simulink model "Train5"  (R2020b)
settings: Solver=VariableStepAuto  StartTime=0.0  StopTime=10.0  RelTol=1e-3
model workspace (MAT data in the model file):
  c = 8
  k = 0.1
undefined symbols (not defined in the file): M_1, M_2, M_3, M_4, M_5, X0_2, X0_3, X0_4, X0_5
settings Model: OrderedModelArguments=off  Creator=zhenya  LastModifiedBy=zhenya

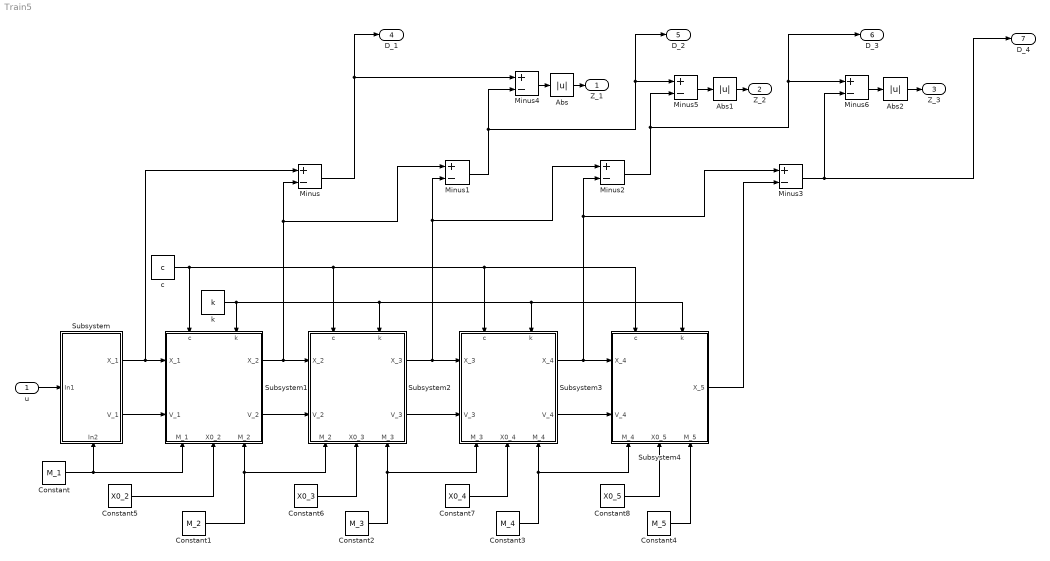
== system Train5 ==
  u : Inport
  Abs : Abs
  Abs1 : Abs
  Abs2 : Abs
  Constant : Constant  Value=M_1
  Constant1 : Constant  Value=M_2
  Constant2 : Constant  Value=M_3
  Constant3 : Constant  Value=M_4
  Constant4 : Constant  Value=M_5
  Constant5 : Constant  Value=X0_2
  Constant6 : Constant  Value=X0_3
  Constant7 : Constant  Value=X0_4
  Constant8 : Constant  Value=X0_5
  Minus{,1..6} (7 alike) : Sum  Inputs=+-
  Subsystem : Subsystem
      settings: PortSchema="{\"entries\":[{\"content\":{\"sides\":[{\"content\":{\"connectorIds\":[\"In1\"]},\"type\":\"ConnectorPlacement.EquallySpacedRectSide\",\"uuid\":\"34ca8425-fccb-4da0-be07-954015c86f74\"},{\"content\":{\"connectorIds\":[\"Out1\",\"Out2\"],\"side\":\"RIGHT\"},\"type\":\"ConnectorPlacement.EquallySpacedRectSide\",\"uuid\":\"a4a70c44-d99b-4f2f-bcd7-1dd85156dc1f\"},{\"content\":{\"connectorIds\":[],\"side\":\"TOP\"},\"type\":\"ConnectorPlacement.EquallySpacedRectSide\",\"uuid\":\"14968497-3b66-4f95-885e-db1a1d92cb6f\"},{\"content\":{\"connectorIds\":[\"In2\"],\"side\":\"BOTTOM\"},\"type\":\"ConnectorPlacement.EquallySpacedRectSide\",\"uuid\":\"7000d41a-f478-4b38-bf4d-e27f7f915c37\"},{\"content\":{\"connectorIds\":[],\"side\":\"HIDDEN\"},\"type\":\"ConnectorPlacement.EquallySpacedRectSide\",\"uuid\":\"79f1d2cd-3fc8-42f6-ae8b-07eaf6f97827\"}]},\"type\":\"ConnectorPlacement.EquallySpacedConnector\",\"uuid\":\"0ff0aa4c-6fa5-4dba-bb7c-396d165f33e0\"}],\"packageUris\":[\"http://schema.mathworks.com/mf0/Connector/R2020b\"],\"version\":\"1.0\"}"
  Subsystem1 : Subsystem
      settings: PortSchema="{\"entries\":[{\"content\":{\"sides\":[{\"content\":{\"connectorIds\":[\"In1\",\"In2\"]},\"type\":\"ConnectorPlacement.EquallySpacedRectSide\",\"uuid\":\"638557b6-12c9-401f-951d-5f98dd7903cc\"},{\"content\":{\"connectorIds\":[\"Out1\",\"Out2\"],\"side\":\"RIGHT\"},\"type\":\"ConnectorPlacement.EquallySpacedRectSide\",\"uuid\":\"d2d0712b-4eed-449a-bee8-cfe81cb0f76e\"},{\"content\":{\"connectorIds\":[\"In3\",\"In4\"],\"side\":\"TOP\"},\"type\":\"ConnectorPlacement.EquallySpacedRectSide\",\"uuid\":\"1558c73d-fb4f-4eb2-a0a5-81154d1cf643\"},{\"content\":{\"connectorIds\":[\"In5\",\"In6\",\"In7\"],\"side\":\"BOTTOM\"},\"type\":\"ConnectorPlacement.EquallySpacedRectSide\",\"uuid\":\"3af12584-476c-4d41-9154-a12458e629fd\"},{\"content\":{\"connectorIds\":[],\"side\":\"HIDDEN\"},\"type\":\"ConnectorPlacement.EquallySpacedRectSide\",\"uuid\":\"cdf596f7-1fd7-4460-9128-df53dc6c9dd6\"}]},\"type\":\"ConnectorPlacement.EquallySpacedConnector\",\"uuid\":\"66e3da69-735a-4605-b465-2e84808dff46\"}],\"packageUris\":[\"http://schema.mathworks.com/mf0/Connector/R2020b\"],\"version\":\"1.0\"}"
  Subsystem2 : Subsystem
      settings: PortSchema="{\"entries\":[{\"content\":{\"sides\":[{\"content\":{\"connectorIds\":[\"In1\",\"In2\"]},\"type\":\"ConnectorPlacement.EquallySpacedRectSide\",\"uuid\":\"638557b6-12c9-401f-951d-5f98dd7903cc\"},{\"content\":{\"connectorIds\":[\"Out1\",\"Out2\"],\"side\":\"RIGHT\"},\"type\":\"ConnectorPlacement.EquallySpacedRectSide\",\"uuid\":\"d2d0712b-4eed-449a-bee8-cfe81cb0f76e\"},{\"content\":{\"connectorIds\":[\"In3\",\"In4\"],\"side\":\"TOP\"},\"type\":\"ConnectorPlacement.EquallySpacedRectSide\",\"uuid\":\"1558c73d-fb4f-4eb2-a0a5-81154d1cf643\"},{\"content\":{\"connectorIds\":[\"In5\",\"In6\",\"In7\"],\"side\":\"BOTTOM\"},\"type\":\"ConnectorPlacement.EquallySpacedRectSide\",\"uuid\":\"3af12584-476c-4d41-9154-a12458e629fd\"},{\"content\":{\"connectorIds\":[],\"side\":\"HIDDEN\"},\"type\":\"ConnectorPlacement.EquallySpacedRectSide\",\"uuid\":\"cdf596f7-1fd7-4460-9128-df53dc6c9dd6\"}]},\"type\":\"ConnectorPlacement.EquallySpacedConnector\",\"uuid\":\"66e3da69-735a-4605-b465-2e84808dff46\"}],\"packageUris\":[\"http://schema.mathworks.com/mf0/Connector/R2020b\"],\"version\":\"1.0\"}"
  Subsystem3 : Subsystem
      settings: PortSchema="{\"entries\":[{\"content\":{\"sides\":[{\"content\":{\"connectorIds\":[\"In1\",\"In2\"]},\"type\":\"ConnectorPlacement.EquallySpacedRectSide\",\"uuid\":\"638557b6-12c9-401f-951d-5f98dd7903cc\"},{\"content\":{\"connectorIds\":[\"Out1\",\"Out2\"],\"side\":\"RIGHT\"},\"type\":\"ConnectorPlacement.EquallySpacedRectSide\",\"uuid\":\"d2d0712b-4eed-449a-bee8-cfe81cb0f76e\"},{\"content\":{\"connectorIds\":[\"In3\",\"In4\"],\"side\":\"TOP\"},\"type\":\"ConnectorPlacement.EquallySpacedRectSide\",\"uuid\":\"1558c73d-fb4f-4eb2-a0a5-81154d1cf643\"},{\"content\":{\"connectorIds\":[\"In5\",\"In6\",\"In7\"],\"side\":\"BOTTOM\"},\"type\":\"ConnectorPlacement.EquallySpacedRectSide\",\"uuid\":\"3af12584-476c-4d41-9154-a12458e629fd\"},{\"content\":{\"connectorIds\":[],\"side\":\"HIDDEN\"},\"type\":\"ConnectorPlacement.EquallySpacedRectSide\",\"uuid\":\"cdf596f7-1fd7-4460-9128-df53dc6c9dd6\"}]},\"type\":\"ConnectorPlacement.EquallySpacedConnector\",\"uuid\":\"66e3da69-735a-4605-b465-2e84808dff46\"}],\"packageUris\":[\"http://schema.mathworks.com/mf0/Connector/R2020b\"],\"version\":\"1.0\"}"
  Subsystem4 : Subsystem
      settings: PortSchema="{\"entries\":[{\"content\":{\"sides\":[{\"content\":{\"connectorIds\":[\"In1\",\"In2\"]},\"type\":\"ConnectorPlacement.EquallySpacedRectSide\",\"uuid\":\"638557b6-12c9-401f-951d-5f98dd7903cc\"},{\"content\":{\"connectorIds\":[\"Out1\"],\"side\":\"RIGHT\"},\"type\":\"ConnectorPlacement.EquallySpacedRectSide\",\"uuid\":\"d2d0712b-4eed-449a-bee8-cfe81cb0f76e\"},{\"content\":{\"connectorIds\":[\"In3\",\"In4\"],\"side\":\"TOP\"},\"type\":\"ConnectorPlacement.EquallySpacedRectSide\",\"uuid\":\"1558c73d-fb4f-4eb2-a0a5-81154d1cf643\"},{\"content\":{\"connectorIds\":[\"In5\",\"In6\",\"In7\"],\"side\":\"BOTTOM\"},\"type\":\"ConnectorPlacement.EquallySpacedRectSide\",\"uuid\":\"3af12584-476c-4d41-9154-a12458e629fd\"},{\"content\":{\"connectorIds\":[],\"side\":\"HIDDEN\"},\"type\":\"ConnectorPlacement.EquallySpacedRectSide\",\"uuid\":\"cdf596f7-1fd7-4460-9128-df53dc6c9dd6\"}]},\"type\":\"ConnectorPlacement.EquallySpacedConnector\",\"uuid\":\"66e3da69-735a-4605-b465-2e84808dff46\"}],\"packageUris\":[\"http://schema.mathworks.com/mf0/Connector/R2020b\"],\"version\":\"1.0\"}"
  c : Constant  Value=c
  k : Constant  Value=k
  Z_1 : Outport
  Z_2 : Outport  Port=2
  Z_3 : Outport  Port=3
  D_1 : Outport  Port=4
  D_2 : Outport  Port=5
  D_3 : Outport  Port=6
  D_4 : Outport  Port=7
  wires:
  u/1 -> Subsystem/1(In1)
  k/1 -> Subsystem4/4(k), Subsystem3/4(k), Subsystem2/4(k), Subsystem1/4(k)
  Constant1/1 -> Subsystem2/5(M_2), Subsystem1/7(M_2)
  Subsystem/2(V_1) -> Subsystem1/2(V_1)
  c/1 -> Subsystem4/3(c), Subsystem3/3(c), Subsystem2/3(c), Subsystem1/3(c)
  Constant/1 -> Subsystem1/5(M_1), Subsystem/2(In2)
  Subsystem1/1(X_2) -> Minus1/1, Minus/2, Subsystem2/1(X_2)
  Subsystem1/2(V_2) -> Subsystem2/2(V_2)
  Constant2/1 -> Subsystem3/5(M_3), Subsystem2/7(M_3)
  Subsystem2/1(X_3) -> Minus1/2, Minus2/1, Subsystem3/1(X_3)
  Subsystem2/2(V_3) -> Subsystem3/2(V_3)
  Constant3/1 -> Subsystem4/5(M_4), Subsystem3/7(M_4)
  Subsystem3/2(V_4) -> Subsystem4/2(V_4)
  Subsystem3/1(X_4) -> Minus3/1, Minus2/2, Subsystem4/1(X_4)
  Constant4/1 -> Subsystem4/7(M_5)
  Subsystem4/1(X_5) -> Minus3/2
  Subsystem/1(X_1) -> Minus/1, Subsystem1/1(X_1)
  Minus/1 -> D_1/1, Minus4/1
  Minus1/1 -> D_2/1, Minus5/1, Minus4/2
  Minus2/1 -> D_3/1, Minus6/1, Minus5/2
  Minus3/1 -> D_4/1, Minus6/2
  Minus4/1 -> Abs/1
  Minus5/1 -> Abs1/1
  Minus6/1 -> Abs2/1
  Abs/1 -> Z_1/1
  Abs1/1 -> Z_2/1
  Abs2/1 -> Z_3/1
  Constant5/1 -> Subsystem1/6(X0_2)
  Constant6/1 -> Subsystem2/6(X0_3)
  Constant7/1 -> Subsystem3/6(X0_4)
  Constant8/1 -> Subsystem4/6(X0_5)

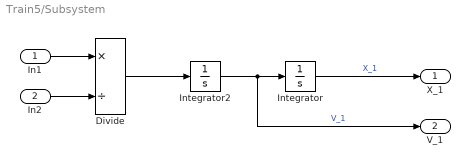
== system Train5/Subsystem ==
  In1 : Inport
  In2 : Inport  Port=2
  Divide : Product  Inputs=*/
  Integrator : Integrator
  Integrator2 : Integrator
  X_1 : Outport
  V_1 : Outport  Port=2
  wires:
  Integrator/1 -> X_1/1  "X_1"
  Integrator2/1 -> V_1/1, Integrator/1  "V_1"
  In1/1 -> Divide/1
  In2/1 -> Divide/2
  Divide/1 -> Integrator2/1

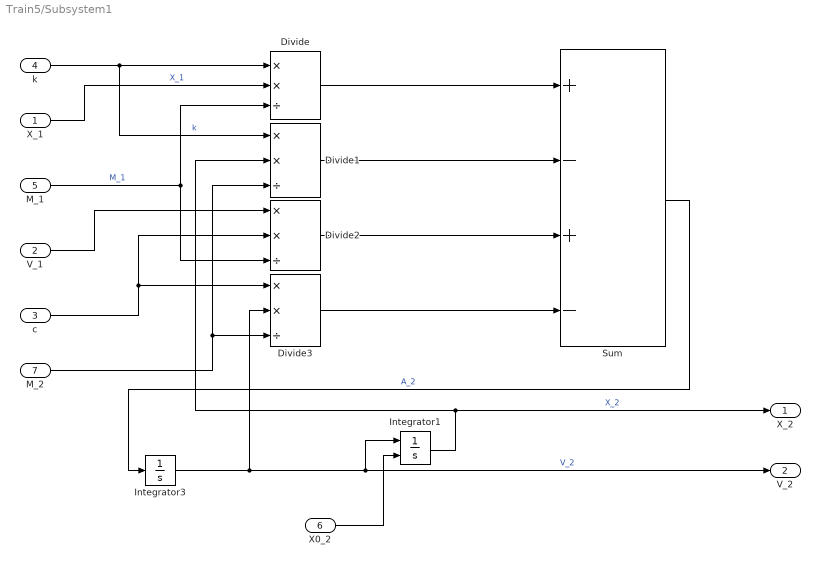
== system Train5/Subsystem1 ==
  X_1 : Inport
  V_1 : Inport  Port=2
  c : Inport  Port=3
  k : Inport  Port=4
  M_1 : Inport  Port=5
  X0_2 : Inport  Port=6
  M_2 : Inport  Port=7
  Divide{,1..3} (4 alike) : Product  Inputs=**/
  Integrator1 : Integrator  InitialConditionSource=external  InitialCondition=-8
  Integrator3 : Integrator
  Sum : Sum  Inputs=+-+-
  X_2 : Outport
  V_2 : Outport  Port=2
  wires:
  Divide2/1 -> Sum/3
  X_1/1 -> Divide/2  "X_1"
  Integrator3/1 -> Integrator1/1, V_2/1, Divide3/2  "V_2"
  Divide1/1 -> Sum/2
  V_1/1 -> Divide2/1
  Divide3/1 -> Sum/4
  Integrator1/1 -> Divide1/2, X_2/1  "X_2"
  Sum/1 -> Integrator3/1  "A_2"
  k/1 -> Divide1/1, Divide/1  "k"
  M_1/1 -> Divide2/3, Divide/3  "M_1"
  Divide/1 -> Sum/1
  M_2/1 -> Divide3/3, Divide1/3
  c/1 -> Divide2/2, Divide3/1
  X0_2/1 -> Integrator1/2

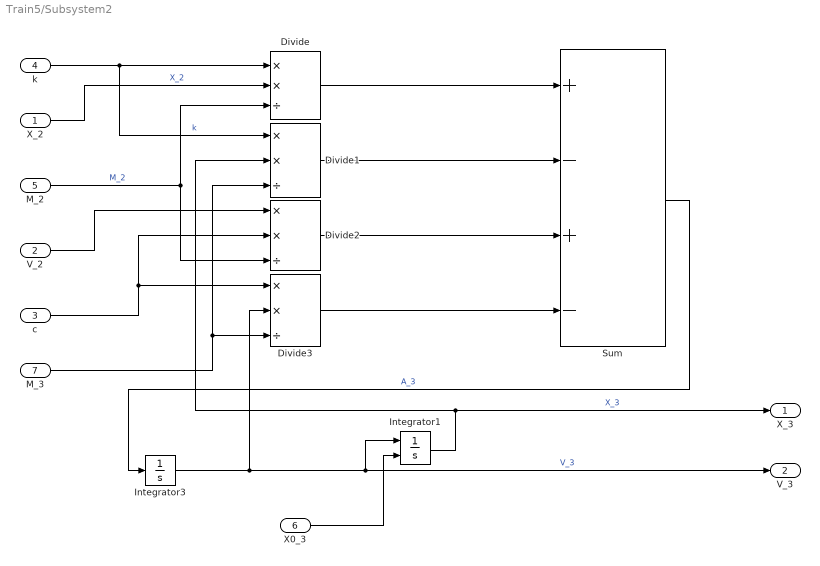
== system Train5/Subsystem2 ==
  X_2 : Inport
  V_2 : Inport  Port=2
  c : Inport  Port=3
  k : Inport  Port=4
  M_2 : Inport  Port=5
  X0_3 : Inport  Port=6
  M_3 : Inport  Port=7
  Divide{,1..3} (4 alike) : Product  Inputs=**/
  Integrator1 : Integrator  InitialConditionSource=external  InitialCondition=-18
  Integrator3 : Integrator
  Sum : Sum  Inputs=+-+-
  X_3 : Outport
  V_3 : Outport  Port=2
  wires:
  Divide2/1 -> Sum/3
  X_2/1 -> Divide/2  "X_2"
  Integrator3/1 -> Integrator1/1, V_3/1, Divide3/2  "V_3"
  Divide1/1 -> Sum/2
  V_2/1 -> Divide2/1
  Divide3/1 -> Sum/4
  Integrator1/1 -> Divide1/2, X_3/1  "X_3"
  Sum/1 -> Integrator3/1  "A_3"
  k/1 -> Divide1/1, Divide/1  "k"
  M_2/1 -> Divide2/3, Divide/3  "M_2"
  Divide/1 -> Sum/1
  M_3/1 -> Divide3/3, Divide1/3
  c/1 -> Divide2/2, Divide3/1
  X0_3/1 -> Integrator1/2

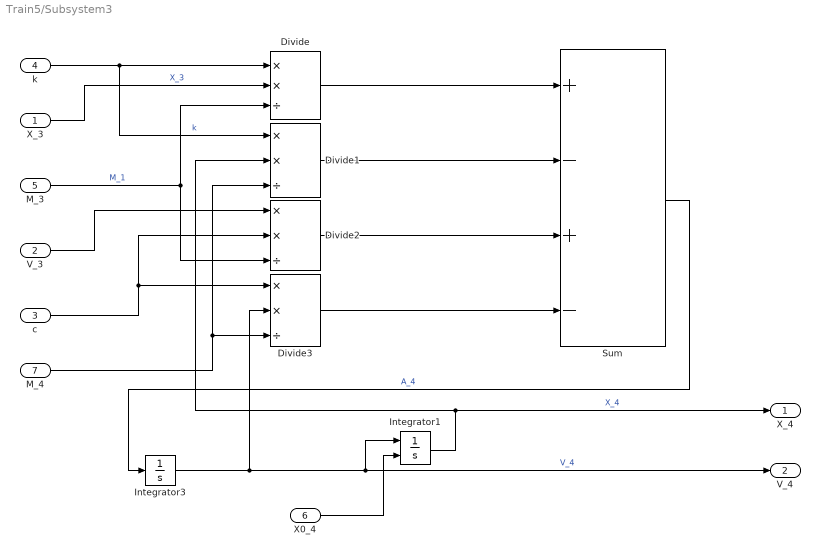
== system Train5/Subsystem3 ==
  X_3 : Inport
  V_3 : Inport  Port=2
  c : Inport  Port=3
  k : Inport  Port=4
  M_3 : Inport  Port=5
  X0_4 : Inport  Port=6
  M_4 : Inport  Port=7
  Divide{,1..3} (4 alike) : Product  Inputs=**/
  Integrator1 : Integrator  InitialConditionSource=external  InitialCondition=-26.2
  Integrator3 : Integrator
  Sum : Sum  Inputs=+-+-
  X_4 : Outport
  V_4 : Outport  Port=2
  wires:
  Divide2/1 -> Sum/3
  X_3/1 -> Divide/2  "X_3"
  Integrator3/1 -> Integrator1/1, V_4/1, Divide3/2  "V_4"
  Divide1/1 -> Sum/2
  V_3/1 -> Divide2/1
  Divide3/1 -> Sum/4
  Integrator1/1 -> Divide1/2, X_4/1  "X_4"
  Sum/1 -> Integrator3/1  "A_4"
  k/1 -> Divide1/1, Divide/1  "k"
  M_3/1 -> Divide2/3, Divide/3  "M_1"
  Divide/1 -> Sum/1
  M_4/1 -> Divide3/3, Divide1/3
  c/1 -> Divide2/2, Divide3/1
  X0_4/1 -> Integrator1/2

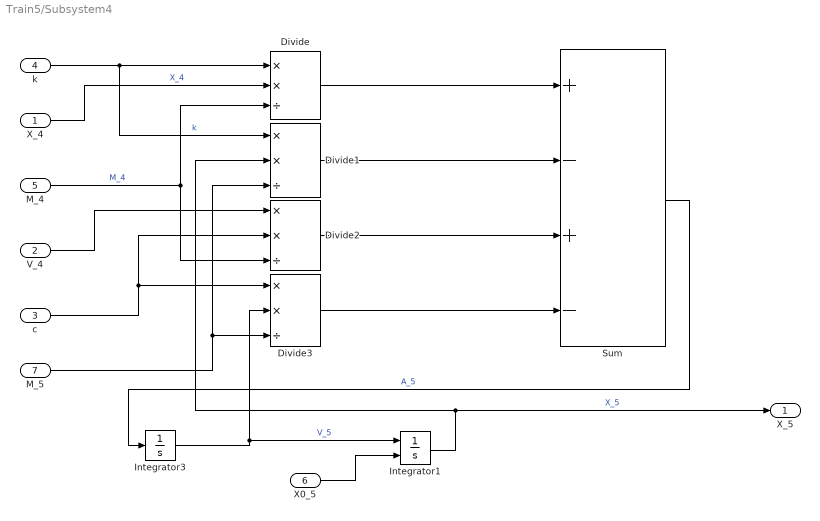
== system Train5/Subsystem4 ==
  X_4 : Inport
  V_4 : Inport  Port=2
  c : Inport  Port=3
  k : Inport  Port=4
  M_4 : Inport  Port=5
  X0_5 : Inport  Port=6
  M_5 : Inport  Port=7
  Divide{,1..3} (4 alike) : Product  Inputs=**/
  Integrator1 : Integrator  InitialConditionSource=external  InitialCondition=-36
  Integrator3 : Integrator
  Sum : Sum  Inputs=+-+-
  X_5 : Outport
  wires:
  Divide2/1 -> Sum/3
  X_4/1 -> Divide/2  "X_4"
  Integrator3/1 -> Integrator1/1, Divide3/2  "V_5"
  Divide1/1 -> Sum/2
  V_4/1 -> Divide2/1
  Divide3/1 -> Sum/4
  Integrator1/1 -> Divide1/2, X_5/1  "X_5"
  Sum/1 -> Integrator3/1  "A_5"
  k/1 -> Divide1/1, Divide/1  "k"
  M_4/1 -> Divide2/3, Divide/3  "M_4"
  Divide/1 -> Sum/1
  M_5/1 -> Divide3/3, Divide1/3
  c/1 -> Divide2/2, Divide3/1
  X0_5/1 -> Integrator1/2
